simulink model "chap1_19"  (Simulink 3.00)
settings: Solver=ode45  StartTime=0.0  StopTime=1.0  RelTol=1e-3
values from neighbouring files (symbols this model uses):
  ki = 2.0    (= 2)    [chap1_10.m]    (also in chap1_12.m = 0.1; chap1_13.m = 0.005; chap1_15.m = 9; chap1_16.m = 0.0048)
  kp = 1.0    (= 1)    [chap1_10.m]    (also in chap1_12.m = 8; chap1_13.m = 0.8; chap1_15.m = 0.85; chap1_16.m = 0.45)
  ts = 0.001    [chap1_10.m]    (also in chap1_12.m; chap1_13.m = 20; chap1_15.m; chap1_16.m = 20)
undefined symbols (not defined in the file or in its folder): den, denQ, num, numQ
libraries: simulink3 x1

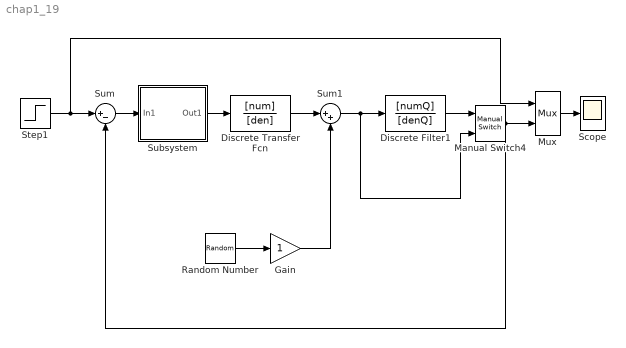
== system chap1_19 ==
  Discrete Transfer Fcn : DiscreteTransferFcn  Numerator=[num]  Denominator=[den]  SampleTime=ts
  Discrete Filter1 : DiscreteFilter  Numerator=[numQ]  Denominator=[denQ]  SampleTime=ts
  Gain : Gain  Gain=1  SaturateOnIntegerOverflow=on
  Manual Switch4 : simulink3/Nonlinear/Manual Switch  sw=0  action=0
  Mux : Mux  Inputs=2
      settings: DisplayOption=none
  Random Number : RandomNumber  Mean=0  Variance=1  Seed=0  SampleTime=ts
  Scope : Scope
      settings: TimeRange=auto  YMin=-5  YMax=5  SaveToWorkspace=off  SaveName=ScopeData
  Step1 : Step  Time=0  Before=0  After=20  SampleTime=ts
  Subsystem : Subsystem
  Sum : Sum  Inputs=|+-  SaturateOnIntegerOverflow=on
  Sum1 : Sum  Inputs=|++  SaturateOnIntegerOverflow=on
  wires:
  Discrete Transfer Fcn/1 -> Sum1/1
  Discrete Filter1/1 -> Manual Switch4/1
  Sum1/1 -> Discrete Filter1/1, Manual Switch4/2
  Subsystem/1(Out1) -> Discrete Transfer Fcn/1
  Mux/1 -> Scope/1
  Manual Switch4/1 -> Sum/2, Mux/2
  Step1/1 -> Sum/1, Mux/1
  Random Number/1 -> Gain/1
  Sum/1 -> Subsystem/1(In1)
  Gain/1 -> Sum1/2

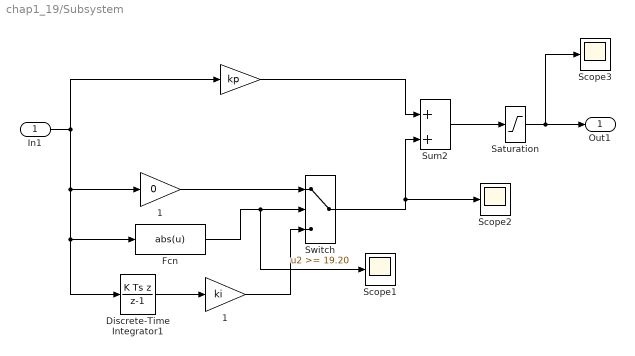
== system chap1_19/Subsystem ==
  In1 : Inport  Port=1  PortWidth=-1  SampleTime=-1  DataType=auto
      settings: SignalType=auto
  "  " : Gain  Gain=kp  SaturateOnIntegerOverflow=on
  "   1" : Gain  Gain=0  SaturateOnIntegerOverflow=on
  " 1" : Gain  Gain=ki  SaturateOnIntegerOverflow=on
  Discrete-Time Integrator1 : DiscreteIntegrator  IntegratorMethod=BackwardEuler  ExternalReset=none  InitialConditionSource=internal  InitialCondition=0  LimitOutput=off  UpperSaturationLimit=inf  LowerSaturationLimit=-inf  ShowSaturationPort=off  ShowStatePort=off  SampleTime=ts
  Fcn : Fcn  Expr=abs(u)
  Saturation : Saturate  UpperLimit=10  LowerLimit=-10
  Scope1 : Scope
      settings: TimeRange=auto  YMin=-5  YMax=5  SaveToWorkspace=off  SaveName=ScopeData
  Scope2 : Scope
      settings: TimeRange=auto  YMin=-5  YMax=5  SaveToWorkspace=off  SaveName=ScopeData
  Scope3 : Scope
      settings: TimeRange=auto  YMin=-5  YMax=5  SaveToWorkspace=off  SaveName=ScopeData
  Sum2 : Sum  Inputs=|++  SaturateOnIntegerOverflow=on
  Switch : Switch  Threshold=19.20
  Out1 : Outport  Port=1
  wires:
  "  "/1 -> Sum2/1
  Sum2/1 -> Saturation/1
  In1/1 -> "  "/1, "   1"/1, Discrete-Time Integrator1/1, Fcn/1
  Discrete-Time Integrator1/1 -> " 1"/1
  "   1"/1 -> Switch/1
  " 1"/1 -> Switch/3
  Fcn/1 -> Switch/2, Scope1/1
  Switch/1 -> Sum2/2, Scope2/1
  Saturation/1 -> Out1/1, Scope3/1
